simulink model "Ctrl_servo"  (R2020a)
settings: Solver=VariableStepAuto  StartTime=0.0  StopTime=30  RelTol=1e-3
libraries: simulink x3
settings Model: Creator=João Fernando Rangel  LastModifiedBy=João Fernando Rangel

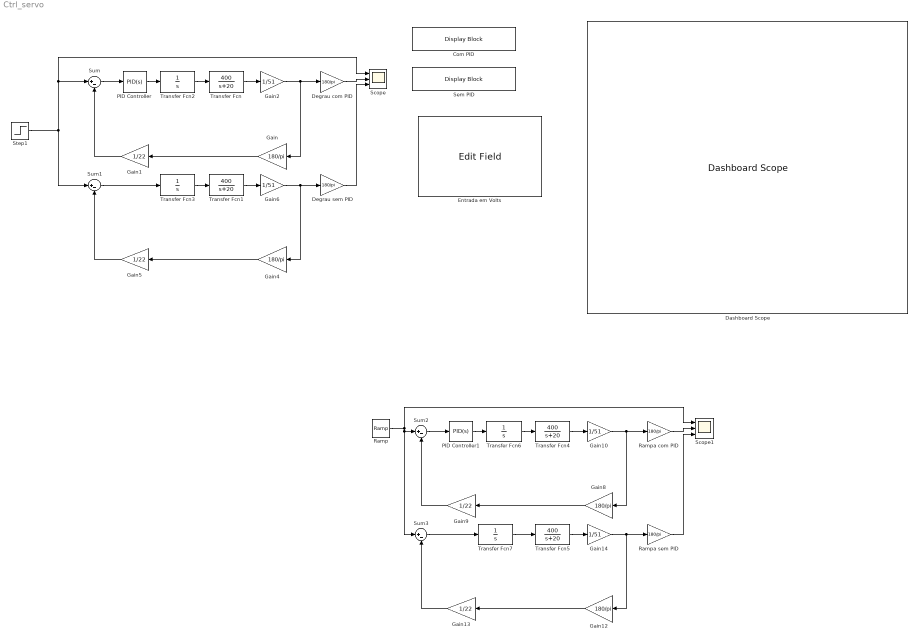
== system Ctrl_servo ==
  Com PID : DisplayBlock  LabelPosition=Hide  Format=short  Transparency=1
  Dashboard Scope : DashboardScope  Ymin=0  Ymax=190
  Degrau com PID : Gain  Gain=180/pi
  Degrau sem PID : Gain  Gain=180/pi
  Entrada em Volts : EditField  LabelPosition=Hide  ShowInitialText=on  Alignment=Center
  Gain{,4,8,12} (4 alike) : Gain  Gain=180/pi
  Gain{1,5,9,13} (4 alike) : Gain  Gain=1/22
  Gain{2,6,10,14} (4 alike) : Gain  Gain=1/51
  PID Controller : simulink/Continuous/PID Controller  Controller=PID  Form=Parallel  TimeDomain=Continuous-time  UseExternalTs=off  SampleTime=-1  IntegratorMethod=Forward Euler  FilterMethod=Forward Euler  ControllerParametersSource=internal  P=37.68  I=76.75  D=1.888  UseFilter=on  N=100  TunerSelectOption=Transfer Function Based (PID Tuner App)  InitialConditionSource=internal  InitialConditionForIntegrator=0  InitialConditionForFilter=0  DifferentiatorICPrevScaledInput=0  ExternalReset=none  TrackingMode=off  Kt=1  LimitOutput=off  UpperSaturationLimit=inf  LowerSaturationLimit=-inf  LinearizeAsGain=on  AntiWindupMode=none  Kb=1  POutMin=[]  POutMax=[]  IOutMin=[]  IOutMax=[]  DOutMin=[]  DOutMax=[]  NOutMin=[]  NOutMax=[]  SumOutMin=[]  SumOutMax=[]  SaturationOutMin=[]  SaturationOutMax=[]  PParamMin=[]  PParamMax=[]  IParamMin=[]  IParamMax=[]  DParamMin=[]  DParamMax=[]  NParamMin=[]  NParamMax=[]  KbParamMin=[]  KbParamMax=[]  KtParamMin=[]  KtParamMax=[]  KbOutMin=[]  KbOutMax=[]  KtOutMin=[]  KtOutMax=[]  IntegratorOutMin=[]  IntegratorOutMax=[]  FilterOutMin=[]  FilterOutMax=[]  SumI1OutMin=[]  SumI1OutMax=[]  SumI2OutMin=[]  SumI2OutMax=[]  SumI3OutMin=[]  SumI3OutMax=[]  SumI4OutMin=[]  SumI4OutMax=[]  SumDOutMin=[]  SumDOutMax=[]  DifferentiatorOutMin=[]  DifferentiatorOutMax=[]  FilterDiffOutCoefMin=[]  FilterDiffOutCoefMax=[]  ReciprocalOutMin=[]  ReciprocalOutMax=[]  SumDenOutMin=[]  SumDenOutMax=[]  SumNumOutMin=[]  SumNumOutMax=[]  DivideOutMin=[]  DivideOutMax=[]  UdiffTsProdOutMin=[]  UdiffTsProdOutMax=[]  NTsProdOutMin=[]  NTsProdOutMax=[]  UintegralTsProdOutMin=[]  UintegralTsProdOutMax=[]  UngainTsProdOutMin=[]  UngainTsProdOutMax=[]  IntegratorContinuousStateAttributes=''  IntegratorStateMustResolveToSignalObject=off  IntegratorRTWStateStorageClass=Auto  FilterContinuousStateAttributes=''  FilterStateMustResolveToSignalObject=off  FilterRTWStateStorageClass=Auto  ParallelPVariant=InternalParameters  IdealPVariant=Disabled  IVariant=InternalParameters  DVariant=InternalParameters  IntegratorVariant=Continuous  SatVariant=Disabled  AWVariant=Passthrough  PCopyVariant=Disabled  TRVariant=Disabled  FdbkBlocksVariant=Forward  IdealPFdbkVariant=Disabled  SatFdbkVariant=Disabled  DerivativeFilterVariant=ContFilter  NVariant=InternalParameters  NCopyVariant=Disabled  FilterICVariant=InternalICsFilter  IntegratorICVariant=InternalICs  ExternalResetVariant=Disabled  TRSumVariant=Passthrough  SumFdbkVariant=Disabled  SumVariant=Sum_PID  TsampFilterVariant=InternalTs  TsampNgainVariant=Passthrough  TsampIntegralVariant=Passthrough
  PID Controller1 : simulink/Continuous/PID Controller  Controller=PID  Form=Parallel  TimeDomain=Continuous-time  UseExternalTs=off  SampleTime=-1  IntegratorMethod=Forward Euler  FilterMethod=Forward Euler  ControllerParametersSource=internal  P=37.68  I=76.75  D=1.888  UseFilter=on  N=100  TunerSelectOption=Transfer Function Based (PID Tuner App)  InitialConditionSource=internal  InitialConditionForIntegrator=0  InitialConditionForFilter=0  DifferentiatorICPrevScaledInput=0  ExternalReset=none  TrackingMode=off  Kt=1  LimitOutput=off  UpperSaturationLimit=inf  LowerSaturationLimit=-inf  LinearizeAsGain=on  AntiWindupMode=none  Kb=1  POutMin=[]  POutMax=[]  IOutMin=[]  IOutMax=[]  DOutMin=[]  DOutMax=[]  NOutMin=[]  NOutMax=[]  SumOutMin=[]  SumOutMax=[]  SaturationOutMin=[]  SaturationOutMax=[]  PParamMin=[]  PParamMax=[]  IParamMin=[]  IParamMax=[]  DParamMin=[]  DParamMax=[]  NParamMin=[]  NParamMax=[]  KbParamMin=[]  KbParamMax=[]  KtParamMin=[]  KtParamMax=[]  KbOutMin=[]  KbOutMax=[]  KtOutMin=[]  KtOutMax=[]  IntegratorOutMin=[]  IntegratorOutMax=[]  FilterOutMin=[]  FilterOutMax=[]  SumI1OutMin=[]  SumI1OutMax=[]  SumI2OutMin=[]  SumI2OutMax=[]  SumI3OutMin=[]  SumI3OutMax=[]  SumI4OutMin=[]  SumI4OutMax=[]  SumDOutMin=[]  SumDOutMax=[]  DifferentiatorOutMin=[]  DifferentiatorOutMax=[]  FilterDiffOutCoefMin=[]  FilterDiffOutCoefMax=[]  ReciprocalOutMin=[]  ReciprocalOutMax=[]  SumDenOutMin=[]  SumDenOutMax=[]  SumNumOutMin=[]  SumNumOutMax=[]  DivideOutMin=[]  DivideOutMax=[]  UdiffTsProdOutMin=[]  UdiffTsProdOutMax=[]  NTsProdOutMin=[]  NTsProdOutMax=[]  UintegralTsProdOutMin=[]  UintegralTsProdOutMax=[]  UngainTsProdOutMin=[]  UngainTsProdOutMax=[]  IntegratorContinuousStateAttributes=''  IntegratorStateMustResolveToSignalObject=off  IntegratorRTWStateStorageClass=Auto  FilterContinuousStateAttributes=''  FilterStateMustResolveToSignalObject=off  FilterRTWStateStorageClass=Auto  ParallelPVariant=InternalParameters  IdealPVariant=Disabled  IVariant=InternalParameters  DVariant=InternalParameters  IntegratorVariant=Continuous  SatVariant=Disabled  AWVariant=Passthrough  PCopyVariant=Disabled  TRVariant=Disabled  FdbkBlocksVariant=Forward  IdealPFdbkVariant=Disabled  SatFdbkVariant=Disabled  DerivativeFilterVariant=ContFilter  NVariant=InternalParameters  NCopyVariant=Disabled  FilterICVariant=InternalICsFilter  IntegratorICVariant=InternalICs  ExternalResetVariant=Disabled  TRSumVariant=Passthrough  SumFdbkVariant=Disabled  SumVariant=Sum_PID  TsampFilterVariant=InternalTs  TsampNgainVariant=Passthrough  TsampIntegralVariant=Passthrough
  Ramp : simulink/Sources/Ramp  slope=1  start=0  InitialOutput=0
  "Rampa com PID " : Gain  Gain=180/pi
  Rampa sem PID : Gain  Gain=180/pi
  Scope : Scope  NumInputPorts=3
  Scope1 : Scope  NumInputPorts=3
  Sem PID : DisplayBlock  LabelPosition=Hide  Format=short  Transparency=1
  Step1 : Step  After=15  SampleTime=0
  Sum{,1..3} (4 alike) : Sum  Inputs=|+-
  Transfer Fcn{,1,4..5} (4 alike) : TransferFcn  Numerator=[0 400]  Denominator=[1 20]
  Transfer Fcn{2..3,6..7} (4 alike) : TransferFcn  Numerator=[0 1]  Denominator=[1 0]
  wires:
  Transfer Fcn/1 -> Gain2/1
  Gain2/1 -> Degrau com PID/1, Gain/1
  Gain/1 -> Gain1/1
  Gain1/1 -> Sum/2
  Sum/1 -> PID Controller/1
  Degrau com PID/1 -> Scope/2
  PID Controller/1 -> Transfer Fcn2/1
  Transfer Fcn1/1 -> Gain6/1
  Gain4/1 -> Gain5/1
  Gain6/1 -> Degrau sem PID/1, Gain4/1
  Gain5/1 -> Sum1/2
  Degrau sem PID/1 -> Scope/3
  Sum1/1 -> Transfer Fcn3/1
  Transfer Fcn2/1 -> Transfer Fcn/1
  Transfer Fcn3/1 -> Transfer Fcn1/1
  Transfer Fcn7/1 -> Transfer Fcn5/1
  Rampa sem PID/1 -> Scope1/3
  Gain14/1 -> Rampa sem PID/1, Gain12/1
  Gain13/1 -> Sum3/2
  Gain12/1 -> Gain13/1
  "Rampa com PID "/1 -> Scope1/2
  Transfer Fcn5/1 -> Gain14/1
  PID Controller1/1 -> Transfer Fcn6/1
  Ramp/1 -> Sum3/1, Sum2/1, Scope1/1
  Transfer Fcn6/1 -> Transfer Fcn4/1
  Gain8/1 -> Gain9/1
  Transfer Fcn4/1 -> Gain10/1
  Gain10/1 -> "Rampa com PID "/1, Gain8/1
  Sum3/1 -> Transfer Fcn7/1
  Sum2/1 -> PID Controller1/1
  Gain9/1 -> Sum2/2
  Step1/1 -> Sum1/1, Scope/1, Sum/1
